simulink subsystem "PvtSubSys_AHBC"  (R2020b)
settings: Solver=VariableStepAuto  StartTime=0.0  StopTime=10.0  RelTol=1e-3
undefined symbols (not defined in the file): P_AHBC_ABS_ENABLE, P_AHBC_DRIVE_DIRECTION_ENABLE, P_AHBC_ESP_ENABLE, P_AHBC_FOG_ENABLE, P_AHBC_FOG_TIME, P_AHBC_HIGHBEAM_ACTIVE_GRACE, P_AHBC_LAT_ACC_ENTER, P_AHBC_LAT_ACC_EXIT, P_AHBC_MAX_ONCOMING_DISTANCE_COUPLE2, P_AHBC_MAX_ONCOMING_DISTANCE_ONE2, P_AHBC_MAX_TAILLIGHT_DISTANCE_COUPLE2, P_AHBC_MAX_TAILLIGHT_DISTANCE_ONE2, P_AHBC_SPEED_SWITCH_HIGH_BEAM_OFF2, P_AHBC_SPEED_SWITCH_HIGH_BEAM_ON2, P_AHBC_TrafficStyle, P_AHBC_TURN_LAMP_ENABLE, P_AHBC_WIPER_ENABLE, P_AHBC_WIPER_TIME, P_AHBC_YAW_RATE_ENTER, P_AHBC_YAW_RATE_EXIT
libraries: simulink x57
(part 4 of 4)

== matlab function PvtSubSys_AHBC/Subsystem1/AHBC/ADB_adapter/MATLAB Function1 ==
  data: LSV_valid_state input uint8; LSR_valid_state input uint8; LSV_ID input uint8; LSV_Is_New input uint8; LSV_Confidence input single; LSV_Consecutive_Detection input int8; LSV_Type input uint8; LSV_Sub_Type input uint8; LSV_CL_Sub_Type input uint8; LSV_Distance input uint16; LSV_Right_Angle input single; LSV_Left_Angle input single; LSV_Top_Angle input single; LSV_Angular_Velocity_Right input single; LSV_Angular_Velocity_Left input single; LSR_ID input uint8; LSR_Distance input uint16; LSR_Right_Angle input single; LSR_Left_Angle input single; LSR_Top_Angle input single; LSV_valid_stateK input uint8; LSV_List output Bus: UserDefined_LSV_ELEM_BUS; LSR_List output Bus: UserDefined_LSR_ELEM_BUS; LSV_ListK input Bus: UserDefined_LSV_ELEM_BUS
% function [LSV_ID1,LSV_Is_New1,LSV_Confidence1,LSV_Consecutive_Detection1,LSV_Type1,LSV_Sub_Type1,LSV_CL_Sub_Type1,LSV_Distance1,LSV_Right_Angle1,LSV_Left_Angle1,LSV_Top_Angle1,LSV_Angular_Velocity_Right1,LSV_Angular_Velocity_Left1,...
%     LSV_ID2,LSV_Is_New2,LSV_Confidence2,LSV_Consecutive_Detection2,LSV_Type2,LSV_Sub_Type2,LSV_CL_Sub_Type2,LSV_Distance2,LSV_Right_Angle2,LSV_Left_Angle2,LSV_Top_Angle2,LSV_Angular_Velocity_Right2,LSV_Angular_Velocity_Left2,...
%     LSV_ID3,LSV_Is_New3,LSV_Confidence3,LSV_Consecutive_Detection3,LSV_Type3,LSV_Sub_Type3,LSV_CL_Sub_Type3,LSV_Distance3,LSV_Right_Angle3,LSV_Left_Angle3,LSV_Top_Angle3,LSV_Angular_Velocity_Right3,LSV_Angular_Velocity_Left3,...
%     LSV_ID4,LSV_Is_New4,LSV_Confidence4,LSV_Consecutive_Detection4,LSV_Type4,LSV_Sub_Type4,LSV_CL_Sub_Type4,LSV_Distance4,LSV_Right_Angle4,LSV_Left_Angle4,LSV_Top_Angle4,LSV_Angular_Velocity_Right4,LSV_Angular_Velocity_Left4,...
%     LSV_ID5,LSV_Is_New5,LSV_Confidence5,LSV_Consecutive_Detection5,LSV_Type5,LSV_Sub_Type5,LSV_CL_Sub_Type5,LSV_Distance5,LSV_Right_Angle5,LSV_Left_Angle5,LSV_Top_Angle5,LSV_Angular_Velocity_Right5,LSV_Angular_Velocity_Left5,...
%     LSV_ID6,LSV_Is_New6,LSV_Confidence6,LSV_Consecutive_Detection6,LSV_Type6,LSV_Sub_Type6,LSV_CL_Sub_Type6,LSV_Distance6,LSV_Right_Angle6,LSV_Left_Angle6,LSV_Top_Angle6,LSV_Angular_Velocity_Right6,LSV_Angular_Velocity_Left6,...
%     LSV_ID7,LSV_Is_New7,LSV_Confidence7,LSV_Consecutive_Detection7,LSV_Type7,LSV_Sub_Type7,LSV_CL_Sub_Type7,LSV_Distance7,LSV_Right_Angle7,LSV_Left_Angle7,LSV_Top_Angle7,LSV_Angular_Velocity_Right7,LSV_Angular_Velocity_Left7,...
%     LSV_ID8,LSV_Is_New8,LSV_Confidence8,LSV_Consecutive_Detection8,LSV_Type8,LSV_Sub_Type8,LSV_CL_Sub_Type8,LSV_Distance8,LSV_Right_Angle8,LSV_Left_Angle8,LSV_Top_Angle8,LSV_Angular_Velocity_Right8,LSV_Angular_Velocity_Left8]=...
%     Sign_Slector(LSV_valid_state,LSR_valid_state,...
%     LSV_ID,LSV_Is_New,LSV_Confidence,LSV_Consecutive_Detection,LSV_Type,LSV_Sub_Type,LSV_CL_Sub_Type,LSV_Distance,LSV_Right_Angle,LSV_Left_Angle,LSV_Top_Angle,LSV_Angular_Velocity_Right,LSV_Angular_Velocity_Left)

function [LSV_List,LSR_List] =...
    Sign_Slector(LSV_valid_state,LSR_valid_state,...
    LSV_ID,LSV_Is_New,LSV_Confidence,LSV_Consecutive_Detection,LSV_Type,LSV_Sub_Type,LSV_CL_Sub_Type,LSV_Distance,LSV_Right_Angle,LSV_Left_Angle,LSV_Top_Angle,LSV_Angular_Velocity_Right,LSV_Angular_Velocity_Left,...
    LSR_ID,LSR_Distance,LSR_Right_Angle,LSR_Left_Angle,LSR_Top_Angle,LSV_valid_stateK,LSV_ListK)

%     LSV_ID1=uint8(0);LSV_Is_New1=uint8(0);LSV_Confidence1=single(0);LSV_Consecutive_Detection1=int8(0);LSV_Type1=uint8(0);LSV_Sub_Type1=uint8(0);LSV_CL_Sub_Type1=uint8(0);LSV_Distance1=uint16(0);LSV_Right_Angle1=single(0);LSV_Left_Angle1=single(0);LSV_Top_Angle1=single(0);LSV_Angular_Velocity_Right1=single(0);LSV_Angular_Velocity_Left1=single(0);
%     LSV_ID2=uint8(0);LSV_Is_New2=uint8(0);LSV_Confidence2=single(0);LSV_Consecutive_Detection2=int8(0);LSV_Type2=uint8(0);LSV_Sub_Type2=uint8(0);LSV_CL_Sub_Type2=uint8(0);LSV_Distance2=uint16(0);LSV_Right_Angle2=single(0);LSV_Left_Angle2=single(0);LSV_Top_Angle2=single(0);LSV_Angular_Velocity_Right2=single(0);LSV_Angular_Velocity_Left2=single(0);
%     LSV_ID3=uint8(0);LSV_Is_New3=uint8(0);LSV_Confidence3=single(0);LSV_Consecutive_Detection3=int8(0);LSV_Type3=uint8(0);LSV_Sub_Type3=uint8(0);LSV_CL_Sub_Type3=uint8(0);LSV_Distance3=uint16(0);LSV_Right_Angle3=single(0);LSV_Left_Angle3=single(0);LSV_Top_Angle3=single(0);LSV_Angular_Velocity_Right3=single(0);LSV_Angular_Velocity_Left3=single(0);
%     LSV_ID4=uint8(0);LSV_Is_New4=uint8(0);LSV_Confidence4=single(0);LSV_Consecutive_Detection4=int8(0);LSV_Type4=uint8(0);LSV_Sub_Type4=uint8(0);LSV_CL_Sub_Type4=uint8(0);LSV_Distance4=uint16(0);LSV_Right_Angle4=single(0);LSV_Left_Angle4=single(0);LSV_Top_Angle4=single(0);LSV_Angular_Velocity_Right4=single(0);LSV_Angular_Velocity_Left4=single(0);
%     LSV_ID5=uint8(0);LSV_Is_New5=uint8(0);LSV_Confidence5=single(0);LSV_Consecutive_Detection5=int8(0);LSV_Type5=uint8(0);LSV_Sub_Type5=uint8(0);LSV_CL_Sub_Type5=uint8(0);LSV_Distance5=uint16(0);LSV_Right_Angle5=single(0);LSV_Left_Angle5=single(0);LSV_Top_Angle5=single(0);LSV_Angular_Velocity_Right5=single(0);LSV_Angular_Velocity_Left5=single(0);
%     LSV_ID6=uint8(0);LSV_Is_New6=uint8(0);LSV_Confidence6=single(0);LSV_Consecutive_Detection6=int8(0);LSV_Type6=uint8(0);LSV_Sub_Type6=uint8(0);LSV_CL_Sub_Type6=uint8(0);LSV_Distance6=uint16(0);LSV_Right_Angle6=single(0);LSV_Left_Angle6=single(0);LSV_Top_Angle6=single(0);LSV_Angular_Velocity_Right6=single(0);LSV_Angular_Velocity_Left6=single(0);
%     LSV_ID7=uint8(0);LSV_Is_New7=uint8(0);LSV_Confidence7=single(0);LSV_Consecutive_Detection7=int8(0);LSV_Type7=uint8(0);LSV_Sub_Type7=uint8(0);LSV_CL_Sub_Type7=uint8(0);LSV_Distance7=uint16(0);LSV_Right_Angle7=single(0);LSV_Left_Angle7=single(0);LSV_Top_Angle7=single(0);LSV_Angular_Velocity_Right7=single(0);LSV_Angular_Velocity_Left7=single(0);
%     LSV_ID8=uint8(0);LSV_Is_New8=uint8(0);LSV_Confidence8=single(0);LSV_Consecutive_Detection8=int8(0);LSV_Type8=uint8(0);LSV_Sub_Type8=uint8(0);LSV_CL_Sub_Type8=uint8(0);LSV_Distance8=uint16(0);LSV_Right_Angle8=single(0);LSV_Left_Angle8=single(0);LSV_Top_Angle8=single(0);LSV_Angular_Velocity_Right8=single(0);LSV_Angular_Velocity_Left8=single(0);


LSV_List_Init=struct(...
    'LSV_ID_Out',{uint8(0),uint8(0),uint8(0),uint8(0),uint8(0),uint8(0)},...
    'LSV_Is_New_Out',{uint8(0),uint8(0),uint8(0),uint8(0),uint8(0),uint8(0)},...
    'LSV_Confidence_Out',{single(0),single(0),single(0),single(0),single(0),single(0)},...
    'LSV_Consecutive_Detection_Out',{int8(0),int8(0),int8(0),int8(0),int8(0),int8(0)},...
    'LSV_Type_Out',{uint8(0),uint8(0),uint8(0),uint8(0),uint8(0),uint8(0)},...
    'LSV_Sub_Type_Out',{uint8(0),uint8(0),uint8(0),uint8(0),uint8(0),uint8(0)},...
    'LSV_CL_Sub_Type_Out',{uint8(0),uint8(0),uint8(0),uint8(0),uint8(0),uint8(0)},...
    'LSV_Distance_Out',{uint16(0),uint16(0),uint16(0),uint16(0),uint16(0),uint16(0)},...
    'LSV_Right_Angle_Out',{single(0),single(0),single(0),single(0),single(0),single(0)},...
    'LSV_Left_Angle_Out',{single(0),single(0),single(0),single(0),single(0),single(0)},...
    'LSV_Top_Angle_Out',{single(0),single(0),single(0),single(0),single(0),single(0)},...
    'LSV_Angular_Velocity_Right_Out',{single(0),single(0),single(0),single(0),single(0),single(0)},...
    'LSV_Angular_Velocity_Left_Out',{single(0),single(0),single(0),single(0),single(0),single(0)});

% LSV_List_0=struct(...
%     'LSV_ID_Out',{uint8(0),uint8(0),uint8(0),uint8(0),uint8(0),uint8(0)},...
%     'LSV_Is_New_Out',{uint8(0),uint8(0),uint8(0),uint8(0),uint8(0),uint8(0)},...
%     'LSV_Confidence_Out',{single(0),single(0),single(0),single(0),single(0),single(0)},...
%     'LSV_Consecutive_Detection_Out',{int8(0),int8(0),int8(0),int8(0),int8(0),int8(0)},...
%     'LSV_Type_Out',{uint8(0),uint8(0),uint8(0),uint8(0),uint8(0),uint8(0)},...
%     'LSV_Sub_Type_Out',{uint8(0),uint8(0),uint8(0),uint8(0),uint8(0),uint8(0)},...
%     'LSV_CL_Sub_Type_Out',{uint8(0),uint8(0),uint8(0),uint8(0),uint8(0),uint8(0)},...
%     'LSV_Distance_Out',{uint16(0),uint16(0),uint16(0),uint16(0),uint16(0),uint16(0)},...
%     'LSV_Right_Angle_Out',{single(0),single(0),single(0),single(0),single(0),single(0)},...
%     'LSV_Left_Angle_Out',{single(0),single(0),single(0),single(0),single(0),single(0)},...
%     'LSV_Top_Angle_Out',{single(0),single(0),single(0),single(0),single(0),single(0)},...
%     'LSV_Angular_Velocity_Right_Out',{single(0),single(0),single(0),single(0),single(0),single(0)},...
%     'LSV_Angular_Velocity_Left_Out',{single(0),single(0),single(0),single(0),single(0),single(0)});




LSR_List_Init=struct(...
    'LSR_ID_Out',{uint8(0),uint8(0)},...
    'LSR_Distance_Out',{uint16(0),uint16(0)},...
    'LSR_Right_Angle_Out',{single(0),single(0)},...
    'LSR_Left_Angle_Out',{single(0),single(0)},...
    'LSR_Top_Angle_Out',{single(0),single(0)});

for i=1:6
    if LSV_valid_state(i)==uint8(1)
        LSV_List_Init(i).LSV_ID_Out=LSV_ID(i);
        LSV_List_Init(i).LSV_Is_New_Out=LSV_Is_New(i);
        LSV_List_Init(i).LSV_Confidence_Out=LSV_Confidence(i);
        LSV_List_Init(i).LSV_Consecutive_Detection_Out=LSV_Consecutive_Detection(i);
        LSV_List_Init(i).LSV_Type_Out=LSV_Type(i);
        LSV_List_Init(i).LSV_Sub_Type_Out=LSV_Sub_Type(i);
        LSV_List_Init(i).LSV_CL_Sub_Type_Out=LSV_CL_Sub_Type(i);
        LSV_List_Init(i).LSV_Distance_Out=LSV_Distance(i);
        LSV_List_Init(i).LSV_Right_Angle_Out=LSV_Right_Angle(i);
        LSV_List_Init(i).LSV_Left_Angle_Out=LSV_Left_Angle(i);
        LSV_List_Init(i).LSV_Top_Angle_Out=LSV_Top_Angle(i);
        LSV_List_Init(i).LSV_Angular_Velocity_Right_Out=LSV_Angular_Velocity_Right(i);
        LSV_List_Init(i).LSV_Angular_Velocity_Left_Out=LSV_Angular_Velocity_Left(i);
    else
        LSV_List_Init(i).LSV_ID_Out=uint8(0);
        LSV_List_Init(i).LSV_Is_New_Out=uint8(0);
        LSV_List_Init(i).LSV_Confidence_Out=single(0);
        LSV_List_Init(i).LSV_Consecutive_Detection_Out=int8(0);
        LSV_List_Init(i).LSV_Type_Out=uint8(0);
        LSV_List_Init(i).LSV_Sub_Type_Out=uint8(0);
        LSV_List_Init(i).LSV_CL_Sub_Type_Out=uint8(0);
        LSV_List_Init(i).LSV_Distance_Out=uint16(0);
        LSV_List_Init(i).LSV_Right_Angle_Out=single(0);
        LSV_List_Init(i).LSV_Left_Angle_Out=single(0);
        LSV_List_Init(i).LSV_Top_Angle_Out=single(0);
        LSV_List_Init(i).LSV_Angular_Velocity_Right_Out=single(0);
        LSV_List_Init(i).LSV_Angular_Velocity_Left_Out=single(0);
    end        
end

for j=1:2
    if LSR_valid_state(j)==uint8(1)
         LSR_List_Init(j).LSR_ID_Out=LSR_ID(j);
         LSR_List_Init(j).LSR_Distance_Out=LSR_Distance(j);
         LSR_List_Init(j).LSR_Right_Angle_Out=LSR_Right_Angle(j);
         LSR_List_Init(j).LSR_Left_Angle_Out=LSR_Left_Angle(j);
         LSR_List_Init(j).LSR_Top_Angle_Out=LSR_Top_Angle(j);   
    else
        LSR_List_Init(j).LSR_ID_Out=uint8(0);
        LSR_List_Init(j).LSR_Distance_Out=uint16(0);
        LSR_List_Init(j).LSR_Right_Angle_Out=single(0);
        LSR_List_Init(j).LSR_Left_Angle_Out=single(0);
        LSR_List_Init(j).LSR_Top_Angle_Out=single(0);
    end
end

LSV_List = LSV_List_Init';
% LSV_List1=LSV_List_Init';
LSR_List=LSR_List_Init';

% for m=1:6
%     for n=1:6
%         if LSV_ListK(m).LSV_ID_Out ~= 0
%             if abs(LSV_List1(n).LSV_Distance_Out - LSV_ListK(m).LSV_Distance_Out)<1.67 &&...
%                 abs(LSV_List1(n).LSV_Left_Angle_Out - LSV_ListK(m).LSV_Left_Angle_Out) < 1.5 && ...
%                  abs(LSV_List1(n).LSV_Right_Angle_Out - LSV_ListK(m).LSV_Right_Angle_Out) < 1.5
%             m_temp = m;
%             n_temp = n;
%                 if m_temp ~= n_temp
%                     LSV_List_temp = LSV_List1(m);
%                     LSV_List1(m) = LSV_List1(n);
%                     LSV_List1(n) = LSV_List_temp;
%                 end
%             end
%         end
%     end
% end
% 
% for q=1:6
%     for p=q+1:6  
%         if LSV_List1(q).LSV_ID_Out ~= 0 && LSV_List1(p).LSV_ID_Out ~= 0
%             if abs(LSV_List1(q).LSV_Distance_Out - LSV_List1(p).LSV_Distance_Out)<1.67 &&...
%                      abs(LSV_List1(q).LSV_Left_Angle_Out - LSV_List1(p).LSV_Left_Angle_Out) < 1.5 && ...
%                      abs(LSV_List1(q).LSV_Right_Angle_Out - LSV_List1(p).LSV_Right_Angle_Out) < 1.5
%             LSV_List1(p).LSV_ID_Out=uint8(0);
%             LSV_List1(p).LSV_Is_New_Out=uint8(0);
%             LSV_List1(p).LSV_Confidence_Out=single(0);
%             LSV_List1(p).LSV_Consecutive_Detection_Out=int8(0);
%             LSV_List1(p).LSV_Type_Out=uint8(0);
%             LSV_List1(p).LSV_Sub_Type_Out=uint8(0);
%             LSV_List1(p).LSV_CL_Sub_Type_Out=uint8(0);
%             LSV_List1(p).LSV_Distance_Out=uint16(0);
%             LSV_List1(p).LSV_Right_Angle_Out=single(0);
%             LSV_List1(p).LSV_Left_Angle_Out=single(0);
%             LSV_List1(p).LSV_Top_Angle_Out=single(0);
%             LSV_List1(p).LSV_Angular_Velocity_Right_Out=single(0);
%             LSV_List1(p).LSV_Angular_Velocity_Left_Out=single(0);
%             end
%         end
%     end
% end
% 
% for j=1:6
%     for k=j+1:6
%         if LSV_List1(j).LSV_ID_Out == 0 && LSV_List1(k).LSV_ID_Out ~= 0
%             LSV_List1(j) = LSV_List1(k);
%             LSV_List1(k).LSV_ID_Out=uint8(0);
%             LSV_List1(k).LSV_Is_New_Out=uint8(0);
%             LSV_List1(k).LSV_Confidence_Out=single(0);
%             LSV_List1(k).LSV_Consecutive_Detection_Out=int8(0);
%             LSV_List1(k).LSV_Type_Out=uint8(0);
%             LSV_List1(k).LSV_Sub_Type_Out=uint8(0);
%             LSV_List1(k).LSV_CL_Sub_Type_Out=uint8(0);
%             LSV_List1(k).LSV_Distance_Out=uint16(0);
%             LSV_List1(k).LSV_Right_Angle_Out=single(0);
%             LSV_List1(k).LSV_Left_Angle_Out=single(0);
%             LSV_List1(k).LSV_Top_Angle_Out=single(0);
%             LSV_List1(k).LSV_Angular_Velocity_Right_Out=single(0);
%             LSV_List1(k).LSV_Angular_Velocity_Left_Out=single(0);
%             break;
%        end
%     end

    
% LSV_List = LSV_List1;
end

== stateflow chart PvtSubSys_AHBC/Subsystem1/AHBC/HMA/HMA_SM ==
  state HMA_OFF
    du:HMA_Sts=0;
    HMA_HibeamReq=0;
  state HMA_ON
    state HMApassive
      du:HMA_Sts=1;HMA_HibeamReq=0;
    state HMAactive
      du:HMA_Sts=2;
      state LaserHighBeamActive
        du:HMA_HibeamReq=2;
      state HighBeamActive
        du:HMA_HibeamReq=1;
      state HighBeamActiveWait
        en:i=0;
        du:i=i+1;
      state LaserHighBeamActiveWait
        en:i=0;
        du:i=i+1;
      state LowBeamActive
        du:HMA_HibeamReq=0;
      HighBeamActive -> LowBeamActive [order 1] : [(HighBeamSuppression...
          | ||(HLB_Decision~=1))...
          | &&~HighPriorityTransformSuppression]
      LaserHighBeamActive -> HighBeamActive [order 2] : [HMA_LaserSuppression...
          | &&VehConfigHMA...
          | &&~HighPriorityTransformSuppression]
      LaserHighBeamActive -> LowBeamActive [order 1] : [(HighBeamSuppression....
          | ||(HLB_Decision~=1))...
          | ||(HMA_LaserSuppression...
          | &&~VehConfigHMA)...
          | &&~HighPriorityTransformSuppression]
      HighBeamActive -> LaserHighBeamActiveWait [order 2] : [~HMA_LaserSuppression...
          | &&VehConfigHMA_laser...
          | &&~HighPriorityTransformSuppression...
          | &&~LowPriorityTransformSuppression]
      HighBeamActiveWait -> HighBeamActive [order 1] : [i>HMA_HIGHBEAM_ACTIVE_GRACE/1000/0.02]
      LaserHighBeamActiveWait -> LaserHighBeamActive [order 1] : [i>HMA_HIGHBEAM_ACTIVE_GRACE/1000/0.02]
      LaserHighBeamActiveWait -> HighBeamActiveWait [order 3] : [HMA_LaserSuppression...
          | &&VehConfigHMA...
          | &&~HighPriorityTransformSuppression]
      HighBeamActiveWait -> LaserHighBeamActiveWait [order 2] : [~HMA_LaserSuppression...
          | &&VehConfigHMA_laser...
          | &&~HighPriorityTransformSuppression...
          | &&~LowPriorityTransformSuppression]
      LowBeamActive -> HighBeamActiveWait [order 2] : [(HLB_Decision==1)...
          | &&~HighBeamSuppression...
          | &&VehConfigHMA...
          | &&~HighPriorityTransformSuppression...
          | &&~LowPriorityTransformSuppression]
      HighBeamActiveWait -> LowBeamActive [order 3] : [(HighBeamSuppression...
          | ||(HLB_Decision~=1))...
          | &&~HighPriorityTransformSuppression]
      LowBeamActive -> LaserHighBeamActiveWait [order 1] : [VehConfigHMA_laser...
          | &&~HighBeamSuppression...
          | &&~HMA_LaserSuppression...
          | &&~HighPriorityTransformSuppression...
          | &&~LowPriorityTransformSuppression...
          | &&(HLB_Decision==1)]
      LaserHighBeamActiveWait -> LowBeamActive [order 2] : [(HighBeamSuppression....
          | ||(HLB_Decision~=1))...
          | ||(HMA_LaserSuppression...
          | &&~VehConfigHMA)...
          | &&~HighPriorityTransformSuppression]
      (default) -> LowBeamActive
    (default) -> HMApassive
    HMApassive -> HMAactive : [HLB_Running_Mode==3||HLB_Running_Mode==2]
    HMAactive -> HMApassive : [HLB_Running_Mode==1]
  state TemporaryFault
    du:HMA_Sts=3;
    HMA_HibeamReq=0;
  state PermanentlyFault
    du:HMA_Sts=4;
    HMA_HibeamReq=0;
  (default) -> HMA_OFF
  HMA_OFF -> HMA_ON : [VehConfigHMA||VehConfigHMA_laser]
  HMA_ON -> HMA_OFF [order 1] : [~VehConfigHMA&&~VehConfigHMA_laser]
  HMA_ON -> TemporaryFault [order 2] : [HMA_Error==1]
  TemporaryFault -> HMA_ON [order 1] : [HMA_Error==0]
  TemporaryFault -> PermanentlyFault [order 2] : [HMA_Error==2]
  HMA_ON -> PermanentlyFault [order 3] : [HMA_Error==2]
  data: VehConfigHMA input uint8; VehConfigHMA_laser input uint8; HMA_Error input uint8; HLB_Running_Mode input uint8; HLB_Decision input uint8; HighBeamSuppression input boolean; HMA_HibeamReq output uint8; LowPriorityTransformSuppression input boolean; HighPriorityTransformSuppression input boolean; HMA_Sts output uint8; HMA_LaserSuppression input boolean; HMA_HIGHBEAM_ACTIVE_GRACE input uint16; i local uint16

== stateflow chart PvtSubSys_AHBC/Subsystem1/AHBC/HMA/HMA_VehSuppression_clc/FodSSclc ==
  state timedelay
    en:i=0;
    du:i=i+1;
  state FogS
    du:FogSS=true;
  state NoFogS
    du:FogSS=false;
  NoFogS -> timedelay : [FFogLmpSts_F_Pbox]
  timedelay -> FogS [order 1] : [i>HMA_FOG_TIME/0.02]
  timedelay -> NoFogS [order 2] : [~FFogLmpSts_F_Pbox]
  FogS -> NoFogS : [~FFogLmpSts_F_Pbox]
  (default) -> NoFogS
  data: FFogLmpSts_F_Pbox input; FogSS output; HMA_FOG_TIME input; i local

== stateflow chart PvtSubSys_AHBC/Subsystem1/AHBC/HMA/HMA_VehSuppression_clc/FodSSclc1 ==
  state timedelay
    en:i=0;
    du:i=i+1;
  state FogS
    du:FogSS=true;
  state NoFogS
    du:FogSS=false;
  NoFogS -> timedelay : [RFogLmpSts__Pbox]
  timedelay -> FogS [order 1] : [i>HMA_FOG_TIME/0.02]
  timedelay -> NoFogS [order 2] : [~RFogLmpSts__Pbox]
  FogS -> NoFogS : [~RFogLmpSts__Pbox]
  (default) -> NoFogS
  data: RFogLmpSts__Pbox input; FogSS output; HMA_FOG_TIME input; i local

== stateflow chart PvtSubSys_AHBC/Subsystem1/AHBC/HMA/HMA_VehSuppression_clc/WiprSSclc ==
  state timedelay
    en:i=0;
    du:i=i+1;
  state WiprS
    du:WiprSS=true;
  state NoWiprS
    du:WiprSS=false;
  NoWiprS -> timedelay : [FrntWiprSwtSts==3 || (FrntWiprSwtSts==1&&WiprReq==3)]
  timedelay -> WiprS [order 1] : [i>HMA_WIPER_TIME/0.02]
  timedelay -> NoWiprS [order 2] : [[~(FrntWiprSwtSts==3 || (FrntWiprSwtSts==1&&WiprReq==3))]]
  WiprS -> NoWiprS : [~(FrntWiprSwtSts==3 || (FrntWiprSwtSts==1&&WiprReq==3))]
  (default) -> NoWiprS
  data: FrntWiprSwtSts input; WiprReq input; HMA_WIPER_TIME input; WiprSS output boolean; i local
